simulink model "LateralController1"  (R2021a)
settings: Solver=VariableStepAuto  StartTime=0.0  StopTime=15  RelTol=1e-3
values from neighbouring files (symbols this model uses):
  CarWidth = 1.4    [controller_setup.m]
  Fyf = zeros(1,57)    [FyfLookup.m]
  ks = 0    [controller_setup.m]    (also in test.m)
  PredictionHorizon = 60    [controller_setup.m]
  SlipAngle = -SlipAngle    [FyfLookup.m]
  Ts = 0.05    [controller_setup.m]    (also in test.m = 0.1)
  Vx = 15    [controller_setup.m]    (also in test.m)
libraries: simulink_extras x4, mpclib x3, simulink x2, autolibshared x1
settings Model: Creator=dekunw  LastModifiedBy=chnwa
settings SolverCC: AlgebraicLoopSolver=TrustRegion
settings DebuggingCC: SFMachineParentedDataDiag=warning

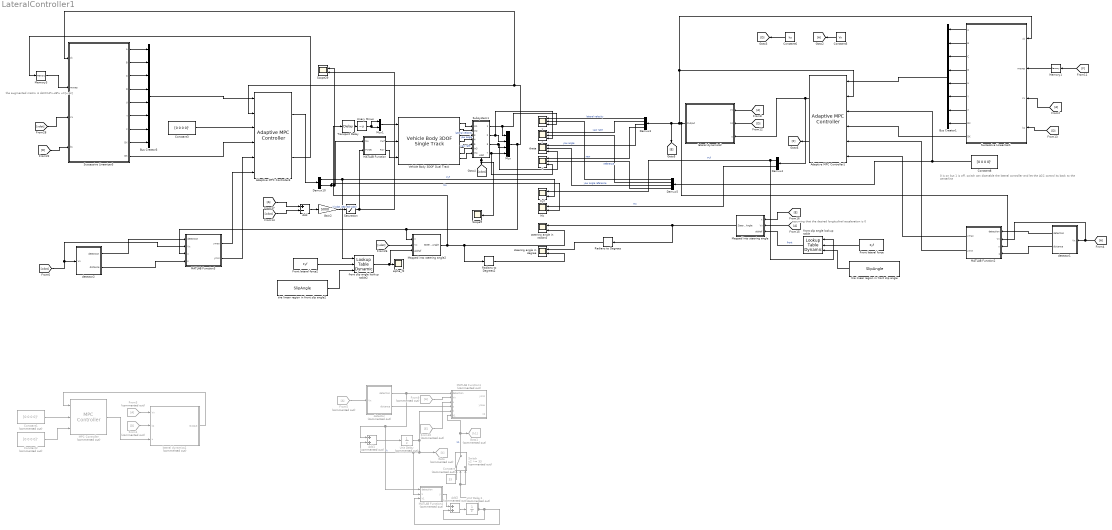
== system LateralController1 ==
  note: 0 is on but 1 is off. switch can disenable the lateral controller and let the ACC control its back to the centerline
  note: assuming that the desired longitudinal acceleration is 0
  note: the augmented matrix is dotX=A*x+B*u
      | u=[u;dc]
  Adaptive MPC Controller1 : mpclib/Adaptive MPC Controller  SCDEnableBlockLinearizationSpecification=on  mpcobj=mpc007  enable_value=0  updateMPCinCallerWorkspace=on  md_inport=on  mv_inport=off  uref_inport=off  return_cost=off  return_mvseq=on  return_qpstatus=off  return_xseq=off  return_state=off  return_ovseq=off  state_inport=off  isltv_plant=on  umin_inport=off  umax_inport=off  ymin_inport=on  ymax_inport=on  cc_inport=off  ywt_inport=off  uwt_inport=off  duwt_inport=off  rhoeps_inport=off  pm_inport=off  MaximumP=10  HorizonChoice=FixedHorizon  BlockDataType=double  SampleTimeInherited=off  switch_inport=off
  Adaptive MPC Controller3 : mpclib/Adaptive MPC Controller  SCDEnableBlockLinearizationSpecification=on  mpcobj=mpc007  enable_value=0  updateMPCinCallerWorkspace=on  md_inport=on  mv_inport=off  uref_inport=off  return_cost=off  return_mvseq=on  return_qpstatus=off  return_xseq=off  return_state=off  return_ovseq=off  state_inport=off  isltv_plant=on  umin_inport=off  umax_inport=off  ymin_inport=on  ymax_inport=on  cc_inport=off  ywt_inport=off  uwt_inport=off  duwt_inport=off  rhoeps_inport=off  pm_inport=off  MaximumP=10  HorizonChoice=FixedHorizon  BlockDataType=double  SampleTimeInherited=off  switch_inport=off
  Add : Sum  Inputs=+-
  Add1 : Sum  Commented=on
  Add2 : Sum  Commented=on
  Bus Creator1 : BusCreator  Inputs=8
  Bus Creator3 : BusCreator  Inputs=8
  Constant : Constant  Commented=on  Value=33
  Constant1 : Constant  Commented=on  Value=[0 0 0 0]'
  Constant2 : Constant  Commented=on  Value=[0 0 0 0]'
  Constant3 : Constant  Value=[0 0 0 0]'
  Constant5 : Constant  Value=Vx
  Constant6 : Constant  Value=ks
  Constant8 : Constant  Value=[0 0 0 0]'
  Demux10 : Demux  Outputs=2
  Demux3 : Demux
  Demux4 : Demux  Outputs=2
  Demux5 : Demux
  From1 : From  Commented=on  GotoTag=D
  From10 : From  Commented=on  GotoTag=E
  From3 : From  Commented=on
  From5 : From  Commented=on
  From9 : From  Commented=on
  Front lateral force : Constant  Value=Fyf
  Front lateral force2 : Constant  Value=Fyf
  Fyf : Scope  NumInputPorts=2
  Gain2 : Gain  Gain=5000
  Goto : Goto  Commented=on  GotoTag=k
  Goto1 : Goto  Commented=on  GotoTag=k1
  MATLAB Function : MATLAB Function  TreatAsAtomicUnit=on
  MATLAB Function1 : MATLAB Function  Commented=on  TreatAsAtomicUnit=on
  MATLAB Function2 : MATLAB Function  TreatAsAtomicUnit=on
  MATLAB Function3 : MATLAB Function  TreatAsAtomicUnit=on
  MATLAB Function4 : MATLAB Function  Commented=on  TreatAsAtomicUnit=on
  MPC Controller : mpclib/MPC Controller  Commented=on  SCDEnableBlockLinearizationSpecification=on  mpcobj=mpc007  is_multiple=0  enable_value=0  return_u0=off  updateMPCinCallerWorkspace=on  md_inport=on  mv_inport=off  uref_inport=off  return_cost=off  return_mvseq=off  return_qpstatus=off  return_xseq=off  return_state=off  return_ovseq=off  state_inport=off  umin_inport=off  umax_inport=off  ymin_inport=off  ymax_inport=off  cc_inport=off  ywt_inport=off  uwt_inport=off  duwt_inport=off  rhoeps_inport=off  pm_inport=off  MaximumP=10  HorizonChoice=FixedHorizon  n_ts=1  n_p=10  n_mv=1  n_md=1  n_ud=0  n_mo=1  n_uo=0  BlockDataType=double  SampleTimeInherited=off  switch_inport=off
  Mapped into steering angle : MATLAB Function  TreatAsAtomicUnit=on
  Mapped into steering angle2 : MATLAB Function  TreatAsAtomicUnit=on
  Memory1 : Memory
  Memory3 : Memory
  Mux : Mux
  Mux1 : Mux  Inputs=2
  Mx : Scope  NumInputPorts=2
  Radians to Degrees : simulink_extras/Transformations/Radians to Degrees
  Radians to Degrees2 : simulink_extras/Transformations/Radians to Degrees
  Saturation : Saturate  UpperLimit=1000  LowerLimit=-1000
  Scope29 : Scope  NumInputPorts=2
  Scope9 : Scope
  Subsystem1 : Subsystem
      settings: PortSchema="{\"entries\":[{\"content\":{\"sides\":[{\"content\":{\"connectorIds\":[\"In1\",\"In2\",\"In3\",\"In4\",\"In5\",\"In6\",\"In7\"]},\"type\":\"ConnectorPlacement.EquallySpacedRectSide\",\"uuid\":\"2d5dd366-cf22-44c4-87a2-f50a57f797af\"},{\"content\":{\"connectorIds\":[\"Out1\",\"Out2\",\"Out3\",\"Out4\"],\"side\":\"RIGHT\"},\"type\":\"ConnectorPlacement.EquallySpacedRectSide\",\"uuid\":\"241189f4-e75c-43e7-8a99-abbcb9c74d53\"},{\"content\":{\"connectorIds\":[],\"side\":\"TOP\"},\"type\":\"ConnectorPlacement.EquallySpacedRectSide\",\"uuid\":\"6b3eeef9-a362-4a78-9c5e-a6ce434eb6a9\"},{\"content\":{\"connectorIds\":[\"Out5\"],\"side\":\"BOTTOM\"},\"type\":\"ConnectorPlacement.EquallySpacedRectSide\",\"uuid\":\"31957e50-4414-4d01-b89b-c25b1ce64d81\"}]},\"type\":\"ConnectorPlacement.EquallySpacedConnector\",\"uuid\":\"717fdc80-cf7e-49a5-b82a-ccb520b44d0e\"}],\"packageUris\":[\"http://schema.mathworks.com/mf0/Connector/R2020b\"],\"version\":\"1.0\"}"
  Successive Linearizer1 : MATLAB Function  TreatAsAtomicUnit=on
  Successive Linearizer3 : MATLAB Function  TreatAsAtomicUnit=on
  Switch : Switch  Commented=on  Threshold=33
  Transport Delay : TransportDelay  DelayTime=Ts
  Unary Minus : UnaryMinus
  Unit Delay : UnitDelay  Commented=on  SampleTime=-1  HasFrameUpgradeWarning=on
  Unit Delay1 : UnitDelay  Commented=on  SampleTime=-1  HasFrameUpgradeWarning=on
  Vehicle Body 3DOF Dual Track : autolibshared/Vehicle Body 3DOF Single Track  trackMode=Dual  inputMode=External longitudinal forces  frontSteerMode=on  rearSteerMode=off  windMode=off  muMode=off  extFMode=off  extMMode=off  htchFMode=off  htchMMode=off  extXo=off  extpsio=off  extxdoto=off  extro=off  extYo=off  extTamb=off  extydoto=off  aMode=2  NF=2  NR=2  m=2272  a=1.11  b=1.67  h=0.35  dh=1  hh=0.2  X_o=0  xdot_o=Vx  CalphaMode=off  sigmaMode=on  d=0  hl=0  w=[CarWidth,CarWidth]  Cy_f=1.3e5  Cy_r=1.28e5  sigma_f=.1  sigma_r=.1  alpha_f_brk=[-.1 .1]  Cy_f_data=[-1.3e5 1.3e5]  alpha_r_brk=[-.1 .1]  Cy_r_data=[-1.3e5 1.3e5]  Y_o=0  ydot_o=0  Izz=4600  psi_o=0  r_o=0  Af=2  Cd=.3  Cl=.1  Cpm=.1  beta_w=[0:0.01:0.3]  Cs=[0:0.03:0.9]  Cym=[0:0.01:0.3]  Pabs=101325  Tair=273  g=9.81  mu=0.7  xdot_tol=.01  Fznom=5000  Fxtire_sat=7e4  Fytire_sat=7e4  longOff=0  latOff=0  vertOff=0  wrapAng=off
      settings: SourceProductBaseCode=PW,DR,MT,UV,VE
  Y : Scope  NumInputPorts=3
  alpha_f2 : Scope
  detector : Subsystem  Commented=on
  detector1 : Subsystem
  detector2 : Subsystem
  front slip angle lookup table : simulink/Lookup Tables/Lookup Table Dynamic  LookUpMeth=Interpolation-Use End Values  OutDataType=fixdt('double')  OutScaling=[]  OutputDataTypeScalingMode=Specify via dialog  OutDataTypeStr=double  DoSatur=off
  front slip angle lookup table2 : simulink/Lookup Tables/Lookup Table Dynamic  LookUpMeth=Interpolation-Use End Values  OutDataType=fixdt('double')  OutScaling=[]  OutputDataTypeScalingMode=Specify via dialog  OutDataTypeStr=double  DoSatur=off
  lateral dynamics1 : Subsystem  Commented=on
  lateral dynamics2 : Subsystem
  r : Scope  NumInputPorts=3
  steering angle in degree : Scope  NumInputPorts=2
  steering angle in radians : Scope  NumInputPorts=2
  theta : Scope  NumInputPorts=3
  tire linear region in front slip angle : Constant  Value=SlipAngle
  tire linear region in front slip angle2 : Constant  Value=SlipAngle
  v : Scope  NumInputPorts=3
  wires:
  Radians to Degrees/1 -> steering angle in degree/1
  Successive Linearizer3/4(D) -> Bus Creator3/4
  Mux/1 -> MATLAB Function3/3(x), Mapped into steering angle2/1(x), Successive Linearizer3/1(xk), Adaptive MPC Controller3/2
  Vehicle Body 3DOF Dual Track/3 -> Subsystem1/3(Input)  "lateral velocity"
  Successive Linearizer3/8(DX) -> Bus Creator3/8
  Vehicle Body 3DOF Dual Track/7 -> Subsystem1/7(In4)
  Vehicle Body 3DOF Dual Track/6 -> Subsystem1/6(In3)
  Adaptive MPC Controller3/2 -> Memory3/1
  Radians to Degrees2/1 -> steering angle in degree/2
  [xdot] -> Mapped into steering angle2/2(Vx)
  Successive Linearizer3/1(A) -> Bus Creator3/1
  Subsystem1/2(Output) -> r/3, Mux/2
  Successive Linearizer3/6(Y) -> Bus Creator3/6
  Gain2/1 -> Saturation/1  "k(xdot_desired-xdot)"
  Successive Linearizer1/8(DX) -> Bus Creator1/8
  Successive Linearizer3/7(X) -> Bus Creator3/7
  [A] -> Mapped into steering angle/2(Vx)
  Successive Linearizer3/2(B) -> Bus Creator3/2
  [D] -> Successive Linearizer3/4(ks)
  From9/1 -> MATLAB Function1/2(Vx)
  Add/1 -> Gain2/1
  tire linear region in front slip angle2/1 -> front slip angle lookup table2/3
  [A] -> Add/1
  Demux10/2 -> Scope29/1, MATLAB Function/1(Mx), Mx/2  "Mx"
  Subsystem1/5(xdot) -> Scope9/1, [xdot]
  [xdot] -> Successive Linearizer3/3(Vx)
  front slip angle lookup table/1 -> Mapped into steering angle/3(alphaf)  "front"
  [xdot] -> Add/2
  Transport Delay/1 -> Unary Minus/1
  Demux3/1 -> v/1  "lateral velocity"
  Constant3/1 -> Adaptive MPC Controller3/3
  Successive Linearizer1/9(DK) -> Adaptive MPC Controller1/4
  Subsystem1/3(Output1) -> theta/3, Mux/3
  Memory3/1 -> Successive Linearizer3/2(moves)
  Successive Linearizer1/7(X) -> Bus Creator1/7
  From10/1 -> MATLAB Function1/3(x)
  Vehicle Body 3DOF Dual Track/5 -> Subsystem1/5(Input2)  "yaw rate"
  Vehicle Body 3DOF Dual Track/2 -> Subsystem1/2(In2)
  Vehicle Body 3DOF Dual Track/1 -> Subsystem1/1(In1)
  Subsystem1/1(Output2) -> Mux/1, v/3
  Constant5/1 -> [A]
  Bus Creator3/1 -> Adaptive MPC Controller3/1
  Adaptive MPC Controller3/1 -> Demux10/1
  [D] -> Successive Linearizer1/4(ks)
  Front lateral force2/1 -> front slip angle lookup table2/2
  Constant6/1 -> [D]
  Demux5/3 -> theta/2  "yaw angle reference"
  Demux5/4 -> Y/2  "reference"
  Demux4/1 -> front slip angle lookup table/1, Fyf/1  "Fyf"
  Front lateral force/1 -> front slip angle lookup table/2
  Vehicle Body 3DOF Dual Track/4 -> Subsystem1/4(Input1)  "yaw angle"
  [E] -> Mapped into steering angle/1(x)
  Adaptive MPC Controller1/1 -> lateral dynamics2/3(u), Demux4/1
  tire linear region in front slip angle/1 -> front slip angle lookup table/3
  Successive Linearizer3/9(DK) -> Adaptive MPC Controller3/4
  Mapped into steering angle/1(SteeringAngle) -> steering angle in radians/1, Radians to Degrees/1
  Adaptive MPC Controller1/2 -> [F]
  Successive Linearizer1/6(Y) -> Bus Creator1/6
  Demux3/2 -> r/1  "yaw rate"
  Mapped into steering angle2/1(SteeringAngle) -> Radians to Degrees2/1, steering angle in radians/2, Transport Delay/1
  [D] -> lateral dynamics2/2(ks)
  Successive Linearizer3/5(U) -> Bus Creator3/5
  Successive Linearizer1/1(A) -> Bus Creator1/1
  Constant8/1 -> Demux5/1, Adaptive MPC Controller1/3
  Successive Linearizer1/3(C) -> Bus Creator1/3
  Successive Linearizer3/3(C) -> Bus Creator3/3
  Bus Creator1/1 -> Adaptive MPC Controller1/1
  Demux3/4 -> Y/1  "new"
  Memory1/1 -> Successive Linearizer1/2(moves)
  [A] -> lateral dynamics2/1(Vx)
  Successive Linearizer1/5(U) -> Bus Creator1/5
  Successive Linearizer1/2(B) -> Bus Creator1/2
  Demux5/2 -> r/2
  lateral dynamics2/1(Output) -> Demux3/1, [E], Successive Linearizer1/1(xk), Adaptive MPC Controller1/2, MATLAB Function2/3(x)
  Successive Linearizer1/4(D) -> Bus Creator1/4
  [F] -> Memory1/1
  Demux5/1 -> v/2
  Demux4/2 -> Mx/1  "Mx"
  [A] -> Successive Linearizer1/3(Vx)
  Demux3/3 -> theta/1  "yaw angle"
  Demux10/1 -> front slip angle lookup table2/1, Fyf/2  "Fyf"
  front slip angle lookup table2/1 -> Mapped into steering angle2/3(alphaf), alpha_f2/1
  MPC Controller/1 -> lateral dynamics1/3(u)
  From1/1 -> lateral dynamics1/2(ks)
  From3/1 -> lateral dynamics1/1(Vx)
  lateral dynamics1/1(Output) -> MPC Controller/1
  Constant1/1 -> MPC Controller/2
  Constant2/1 -> MPC Controller/3
  detector/1(detection) -> MATLAB Function4/1(detection), Add1/1, MATLAB Function1/1(detection)
  detector/2(distance) -> MATLAB Function1/4(s)
  From5/1 -> detector/1(Vx)
  Add1/1 -> Unit Delay/1
  Unit Delay/1 -> MATLAB Function1/5(k), MATLAB Function4/2(k), Add1/2, Goto/1  "k"
  MATLAB Function4/1(y) -> Add2/1
  Add2/1 -> Unit Delay1/1
  Unit Delay1/1 -> Switch/3, Switch/2, MATLAB Function4/3(k1), Add2/2
  Switch/1 -> Goto1/1, MATLAB Function1/6(k1)  "k1"
  Constant/1 -> Switch/1
  [A] -> MATLAB Function2/2(Vx), detector1/1(Vx)
  detector2/2(distance) -> MATLAB Function3/4(s)
  detector2/1(detection) -> MATLAB Function3/1(detection)
  [xdot] -> MATLAB Function3/2(Vx), detector2/1(Vx)
  MATLAB Function3/2(ymin) -> Adaptive MPC Controller3/5
  MATLAB Function3/1(ymax) -> Adaptive MPC Controller3/6
  MATLAB Function2/1(ymax) -> Adaptive MPC Controller1/6
  MATLAB Function2/2(ymin) -> Adaptive MPC Controller1/5
  detector1/2(distance) -> MATLAB Function2/4(s)
  detector1/1(detection) -> MATLAB Function2/1(detection)
  MATLAB Function/1(Fwf) -> Vehicle Body 3DOF Dual Track/2
  MATLAB Function/2(Fwr) -> Vehicle Body 3DOF Dual Track/3
  Mux1/1 -> Vehicle Body 3DOF Dual Track/1
  Subsystem1/4(Y) -> Y/3, Mux/4
  Saturation/1 -> MATLAB Function/2(Fxnet), Scope29/2
  Unary Minus/1 -> Mux1/2, Mux1/1

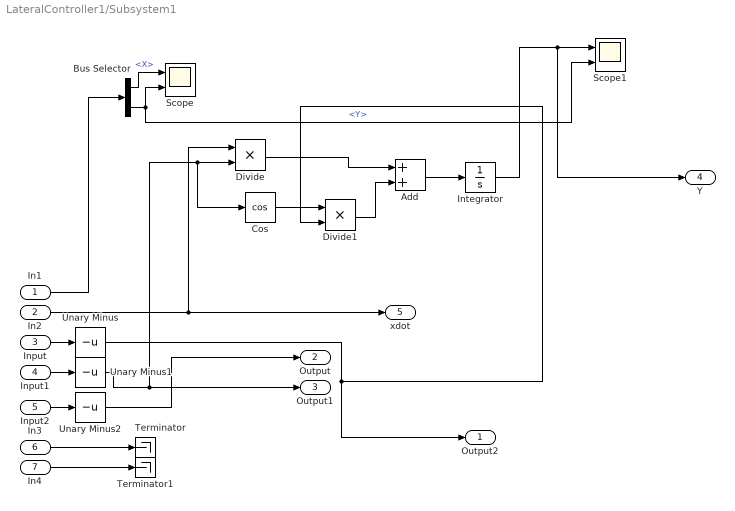
== system LateralController1/Subsystem1 ==
  In1 : Inport
  In2 : Inport  Port=2
  Input : Inport  Port=3
  Input1 : Inport  Port=4
  Input2 : Inport  Port=5
  In3 : Inport  Port=6
  In4 : Inport  Port=7
  Add : Sum
  Bus Selector : BusSelector  OutputSignals=InertFrm.Cg.Disp.X,InertFrm.Cg.Disp.Y
  Cos : Trigonometry  Operator=cos
  Divide : Product  Inputs=**
  Divide1 : Product  Inputs=**
  Integrator : Integrator
  Scope : Scope  NumInputPorts=2
  Scope1 : Scope  NumInputPorts=2
  Terminator : Terminator
  Terminator1 : Terminator
  Unary Minus : UnaryMinus
  Unary Minus1 : UnaryMinus
  Unary Minus2 : UnaryMinus
  Output2 : Outport
  Output : Outport  Port=2
  Output1 : Outport  Port=3
  Y : Outport  Port=4  SampleTime=Ts
  xdot : Outport  Port=5
  wires:
  In4/1 -> Terminator1/1
  In3/1 -> Terminator/1
  In2/1 -> xdot/1, Divide/1
  In1/1 -> Bus Selector/1
  Cos/1 -> Divide1/1
  Divide/1 -> Add/1
  Divide1/1 -> Add/2
  Add/1 -> Integrator/1
  Bus Selector/1 -> Scope/1  "<X>"
  Bus Selector/2 -> Scope/2, Scope1/2  "<Y>"
  Input2/1 -> Unary Minus2/1
  Integrator/1 -> Y/1, Scope1/1
  Input/1 -> Unary Minus/1
  Input1/1 -> Unary Minus1/1
  Unary Minus/1 -> Output2/1, Divide1/2
  Unary Minus1/1 -> Output1/1, Cos/1, Divide/2
  Unary Minus2/1 -> Output/1

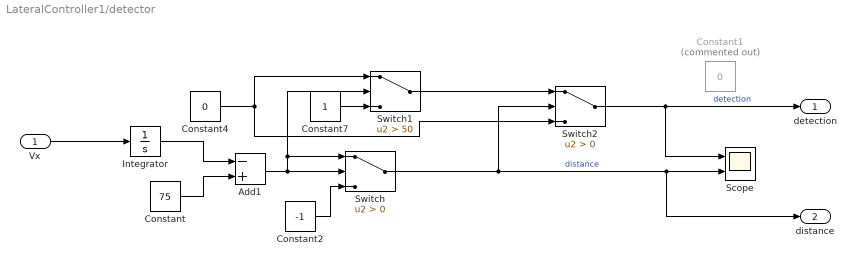
== system LateralController1/detector ==
  Vx : Inport
  Add1 : Sum  Inputs=-+
  Constant : Constant  Value=75
  Constant1 : Constant  Commented=on  Value=0
  Constant2 : Constant  Value=-1
  Constant4 : Constant  Value=0
  Constant7 : Constant
  Integrator : Integrator
  Scope : Scope  NumInputPorts=2
  Switch : Switch  Criteria=u2 > Threshold
  Switch1 : Switch  Criteria=u2 > Threshold  Threshold=50
  Switch2 : Switch  Criteria=u2 > Threshold
  detection : Outport
  distance : Outport  Port=2
  wires:
  Constant2/1 -> Switch/3
  Constant4/1 -> Switch2/3, Switch1/1
  Vx/1 -> Integrator/1
  Integrator/1 -> Add1/1
  Switch/1 -> Switch2/2, distance/1, Scope/2  "distance"
  Constant7/1 -> Switch1/3
  Add1/1 -> Switch1/2, Switch/1, Switch/2
  Switch1/1 -> Switch2/1
  Constant/1 -> Add1/2
  Switch2/1 -> detection/1, Scope/1  "detection"

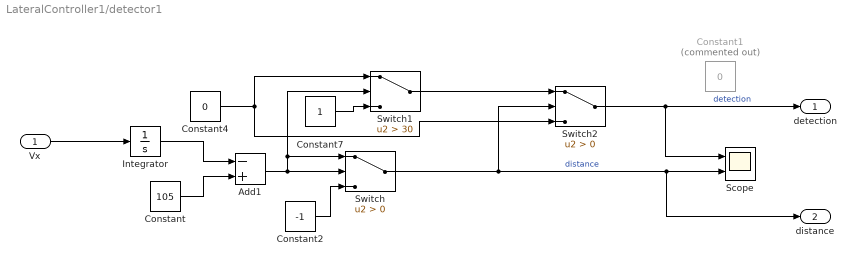
== system LateralController1/detector1 ==
  Vx : Inport
  Add1 : Sum  Inputs=-+
  Constant : Constant  Value=105
  Constant1 : Constant  Commented=on  Value=0
  Constant2 : Constant  Value=-1
  Constant4 : Constant  Value=0
  Constant7 : Constant
  Integrator : Integrator
  Scope : Scope  NumInputPorts=2
  Switch : Switch  Criteria=u2 > Threshold
  Switch1 : Switch  Criteria=u2 > Threshold  Threshold=30
  Switch2 : Switch  Criteria=u2 > Threshold
  detection : Outport
  distance : Outport  Port=2
  wires:
  Constant2/1 -> Switch/3
  Constant4/1 -> Switch2/3, Switch1/1
  Vx/1 -> Integrator/1
  Integrator/1 -> Add1/1
  Switch/1 -> Switch2/2, distance/1, Scope/2  "distance"
  Constant7/1 -> Switch1/3
  Add1/1 -> Switch1/2, Switch/1, Switch/2
  Switch1/1 -> Switch2/1
  Constant/1 -> Add1/2
  Switch2/1 -> Scope/1, detection/1  "detection"

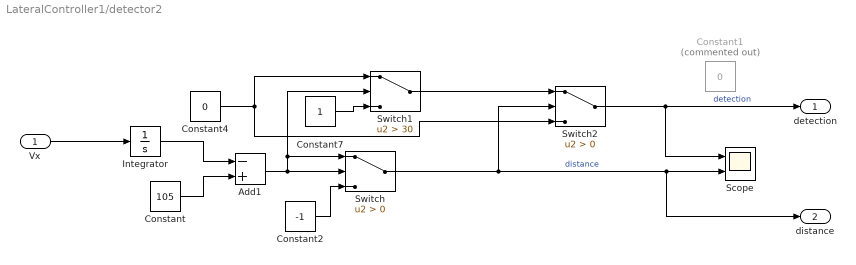
== system LateralController1/detector2 ==
  Vx : Inport
  Add1 : Sum  Inputs=-+
  Constant : Constant  Value=105
  Constant1 : Constant  Commented=on  Value=0
  Constant2 : Constant  Value=-1
  Constant4 : Constant  Value=0
  Constant7 : Constant
  Integrator : Integrator
  Scope : Scope  NumInputPorts=2
  Switch : Switch  Criteria=u2 > Threshold
  Switch1 : Switch  Criteria=u2 > Threshold  Threshold=30
  Switch2 : Switch  Criteria=u2 > Threshold
  detection : Outport
  distance : Outport  Port=2
  wires:
  Constant2/1 -> Switch/3
  Constant4/1 -> Switch2/3, Switch1/1
  Vx/1 -> Integrator/1
  Integrator/1 -> Add1/1
  Switch/1 -> Switch2/2, distance/1, Scope/2  "distance"
  Constant7/1 -> Switch1/3
  Add1/1 -> Switch1/2, Switch/1, Switch/2
  Switch1/1 -> Switch2/1
  Constant/1 -> Add1/2
  Switch2/1 -> Scope/1, detection/1  "detection"

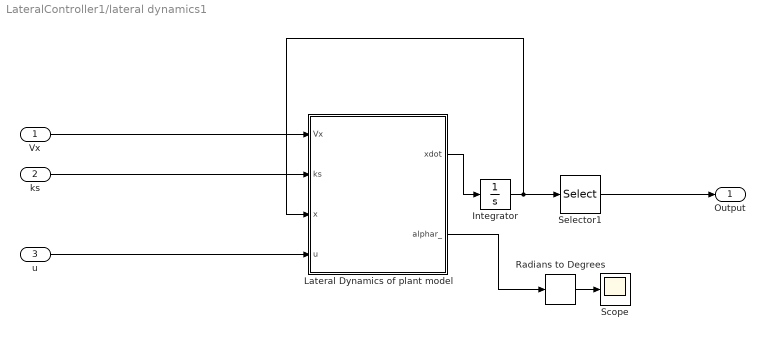
== system LateralController1/lateral dynamics1 ==
  Vx : Inport
  ks : Inport  Port=2
  u : Inport  Port=3
  Integrator : Integrator
  Lateral Dynamics of plant model : MATLAB Function  TreatAsAtomicUnit=on
  Radians to Degrees : simulink_extras/Transformations/Radians to Degrees
  Scope : Scope
  Selector1 : Selector  InputPortWidth=4  IndexOptions=Index vector (dialog)  Indices=[1 2 3 4]  OutputSizes=1
  Output : Outport
  wires:
  u/1 -> Lateral Dynamics of plant model/4(u)
  Lateral Dynamics of plant model/1(xdot) -> Integrator/1
  Integrator/1 -> Selector1/1, Lateral Dynamics of plant model/3(x)
  Selector1/1 -> Output/1
  ks/1 -> Lateral Dynamics of plant model/2(ks)
  Vx/1 -> Lateral Dynamics of plant model/1(Vx)
  Lateral Dynamics of plant model/2(alphar_) -> Radians to Degrees/1
  Radians to Degrees/1 -> Scope/1

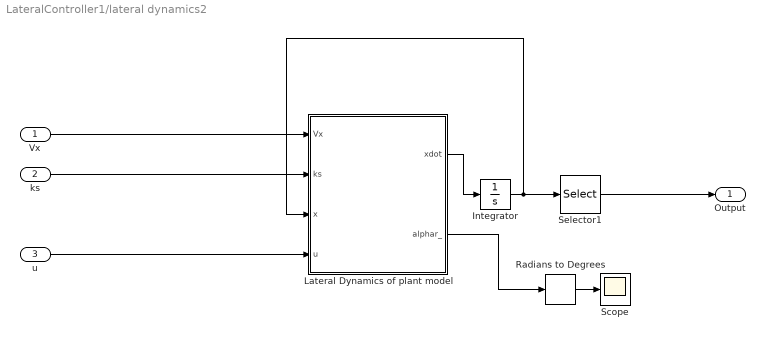
== system LateralController1/lateral dynamics2 ==
  Vx : Inport
  ks : Inport  Port=2
  u : Inport  Port=3
  Integrator : Integrator
  Lateral Dynamics of plant model : MATLAB Function  TreatAsAtomicUnit=on
  Radians to Degrees : simulink_extras/Transformations/Radians to Degrees
  Scope : Scope
  Selector1 : Selector  InputPortWidth=4  IndexOptions=Index vector (dialog)  Indices=[1 2 3 4]  OutputSizes=1
  Output : Outport
  wires:
  u/1 -> Lateral Dynamics of plant model/4(u)
  Lateral Dynamics of plant model/1(xdot) -> Integrator/1
  Integrator/1 -> Selector1/1, Lateral Dynamics of plant model/3(x)
  Selector1/1 -> Output/1
  ks/1 -> Lateral Dynamics of plant model/2(ks)
  Vx/1 -> Lateral Dynamics of plant model/1(Vx)
  Lateral Dynamics of plant model/2(alphar_) -> Radians to Degrees/1
  Radians to Degrees/1 -> Scope/1

== matlab function LateralController1/MATLAB Function4 ==
  data: detection input; y output; k input; k1 input
function y = fcn(detection,k, k1)

if (detection==0)&&(k==33)&&(k1<=33)
    y=1;
else
    y=0;
end

== matlab function LateralController1/Mapped into steering angle ==
  data: x input; Vx input; alphaf input; SteeringAngle output
function SteeringAngle = fcn(x,Vx, alphaf)

lf = 1.11;  % distance from front axle to the mass center

Vy = x(1); %lateral velocity
r = x(2);  %yaw rate
SteeringAngle = Vy/Vx+lf*r/Vx-alphaf;

== matlab function LateralController1/Mapped into steering angle2 ==
  data: x input; Vx input; alphaf input; SteeringAngle output
function SteeringAngle = fcn(x,Vx, alphaf)

lf = 1.11;  % distance from front axle to the mass center

Vy = x(1); %lateral velocity
r = x(2);  %yaw rate
SteeringAngle = Vy/Vx+lf*r/Vx-alphaf;

== matlab function LateralController1/Successive Linearizer3 ==
  data: A output size=[4,4,PredictionHorizon+1]; xk input size=[4,1]; moves input; B output size=[4,6,PredictionHorizon+1]; C output size=[4,4,PredictionHorizon+1]; D output size=[4,6,PredictionHorizon+1]; U output size=[6,1,PredictionHorizon+1]; Y output size=[4,1,PredictionHorizon+1]; X output size=[4,1,PredictionHorizon+1]; DX output size=[4,1,PredictionHorizon+1]; Vx input size=1; ks input; PredictionHorizon parameter size=1; DK output; Ts parameter size=1
function [A,B,C,D,U,Y,X,DX,DK] = fcn(xk,moves,Vx,ks, PredictionHorizon, Ts)
%sucessive updates the LTI plant model required by adaptive MPC controller

% LTV MPC requires p+1 linearizations from k to k+p
Steps = PredictionHorizon + 1; % having the number of Steps models
% Initialize outputs
A = zeros(4,4,Steps);
B = zeros(4,6,Steps);
C = zeros(4,4,Steps);
D = zeros(4,6,Steps);
U = zeros(6,1,Steps);
Y = zeros(4,1,Steps);
X = zeros(4,1,Steps);
DX = zeros(4,1,Steps);
DK = zeros(Steps,4); % the constant matrix in the model considered as measured disturbance

% Obtain time varying linear models via successive linearization
for ct = 1:Steps
    % since we don't have u(k) ... u(k+p) at the time of linearization,
    % previous optimal sequence u(k-1) ... u(k+p-1) is used instead.
    if ct>length(moves)
        uk = moves(Steps,:);
    else
        uk = moves(ct,:);
    end
    uk = uk';
    % analytical linearization (continuous time)
    [Ac, Bc, Cc, Dc, dc] = LateralDynamicsCT(Vx,ks,xk); % acquiring new characteristic matrix
    % convert A and B matrices from continuous time to discrete time
    % augmenting the model to be in the form of dotX=A*x+B*u while u=[u;dc]
    Aca = Ac;
    Bca = [Bc eye(4)];
    M = expm([[Aca Bca zeros(4,1)]*Ts;zeros(7,11)]);
    Ak = M(1:4,1:4);    %the discrete matrix A for augmented model
    Bk = M(1:4,5:10);   %the discrete matrix B for augmented model
    %store the state space matrix for ct time step
    A(:,:,ct) = Ak;
    B(:,:,ct) = Bk;
    C(:,:,ct) = Cc;
    D(:,:,ct) = [Dc,zeros(4,4)];  % always be zeros(4,6) in fact
    U(:,:,ct) = [uk;dc];          % measured disturbance dc is input as well
    Y(:,:,ct) = xk;               % output is all of the four states
    X(:,:,ct) = xk;               % four states
    DX(:,:,ct) = Ak*xk+Bk*[uk;dc]-xk;%the states increment
    DK(ct,:) = dc';               % disturbance in this step
    % next prediction step
    xk = DX(:,:,ct)+xk;           %update the states
end

%%%unrelated stuff
% ct= LTVu15_dist_Ts01.Model.Plant;
% dt = c2d(ct,Ts);
% LTVu15_dist_Ts01.Model.Plant = dt;

== matlab function LateralController1/MATLAB Function ==
  data: Fwf output size=[2,1]; Mx input; Fwr output size=[2,1]; Fxnet input
function [Fwf,Fwr] = fcn(Mx,Fxnet)

w = 1.4; % the width of the car

Fwf = zeros(2,1);
Fwr = zeros(2,1);

if Mx > 0
    Fwf(1) = Fxnet/2-Mx/w;
    Fwf(2) = Fxnet/2+0;
    Fwr(1) = -Mx/w;
    Fwr(2) = 0;
elseif Mx < 0
    Fwf(1) = Fxnet/2+0;
    Fwf(2) = Fxnet/2+Mx/w;
    Fwr(1) = 0;
    Fwr(2) = Mx/w;
else
    Fwf(1) = Fxnet/2+0;
    Fwf(2) = Fxnet/2+0;
    Fwr(1) = 0;
    Fwr(2) = 0;
end

== matlab function LateralController1/lateral dynamics1/Lateral Dynamics of plant model ==
  data: Vx input; ks input; x input; u input; xdot output; alphar_ output
function [xdot,alphar_] = fcn(Vx,ks, x, u)

%Plant Model parameters
m = 2272;   %mass
Iz = 4600;  %rotational inertia
lf = 1.11;  % distance from front axle to the mass center
lr = 1.67;  % distance from rear axle to the mass center
C_a = 1.3e5; % rear cornering stifness 

%Enviroment parameters
miu = 0.7; %frction cooeficient 0.7 for dry road and 0.4 for wet
g = 9.81; % gravity

Fz = m*g*lf/(lf+lr); % the load that beared by the rear tire

%calculate alpha
Vy = x(1); %lateral velocity
r = x(2);  %yaw rate
alphar_ = Vy/Vx-lr*r/Vx;   %calculate linearzing point

%tire model
threshold = atan(3*miu*Fz/C_a);
if abs(alphar_)<threshold
    Fyr_ = -C_a*tan(alphar_)+C_a^2/(3*miu*Fz)*abs(tan(alphar_))*tan(alphar_)-C_a^3/(27*miu^2*Fz^2)*tan(alphar_)^3;
    if alphar_>= 0
        Cr_ = -C_a*sec(alphar_)^2+C_a^2/(3*miu*Fz)*(2*sec(alphar_)^2*tan(alphar_))-C_a^3/(27*miu^2*Fz^2)*(3*tan(alphar_)^2*sec(alphar_)^2);
    else
        Cr_ = -C_a*sec(alphar_)^2-C_a^2/(3*miu*Fz)*(2*sec(alphar_)^2*tan(alphar_))-C_a^3/(27*miu^2*Fz^2)*(3*tan(alphar_)^2*sec(alphar_)^2);
    end
else
    Fyr_ = -miu*Fz*sign(alphar_);
    Cr_ = 0;
end

%Continuous-time model
Ac = [Cr_/(m*Vx) -lr*Cr_/(m*Vx)-Vx 0 0;
    -lr*Cr_/(Iz*Vx) lr^2*Cr_/(Iz*Vx) 0 0;
    0 1 0 0;
    1 0 Vx 0];
Bc = [1/m 0;
    lf/Iz 1/Iz;
    0 0;
    0 0];
dcc = [(Fyr_-Cr_*alphar_)/m;
    -lr*(Fyr_-Cr_*alphar_)/Iz;
    -Vx*ks;
    0];

% Cc =eye(4);
% Dc =zeros(4,2);
xdot = Ac*x + Bc*u +dcc;
% y = C*x + D*u;

== matlab function LateralController1/MATLAB Function2 ==
  data: detection input; ymax output size=[PredictionHorizon,4]; Vx input size=1; x input size=[4,1]; s input; PredictionHorizon parameter; ymin output size=[PredictionHorizon,4]; Ts parameter
function [ymax, ymin] = fcn(detection,Vx,x,s, PredictionHorizon, Ts)

miu = 0.7; %frction cooeficient 0.7 for dry road and 0.4 for wet
g = 9.81; % gravity
m = 2272;   %mass
lf = 1.11;  % distance from front axle to the mass center
lr = 1.67;  % distance from rear axle to the mass center
C_a = 1.3e5; % rear cornering stifness

Fz = m*g*lf/(lf+lr); % the load that beared by the rear tire

rmax = g*miu/Vx; %max yaw rate
threshold = atan(3*miu*Fz/C_a);

r = x(2);
vmax = lr*r+Vx*threshold;   %max lateral velocity
vmin = lr*r-Vx*threshold;   %min lateral velocity
k = round(s/Vx/Ts);
if k>PredictionHorizon
    k =PredictionHorizon;
elseif k<20
    k=20;
end

if detection == 1
    ymin1 = [vmin -rmax -pi/2 -10];%50m is the distance from which obstacle is detected
    ymax1 = [vmax rmax pi/2 10];
    ymin = repmat(ymin1,PredictionHorizon,1);
    ymax = repmat(ymax1,PredictionHorizon,1);
    k1=k-round(3/Vx/Ts);
    k2=k+round(3/Vx/Ts);
    if k1<1
        k1=1;
    end
    if k2>PredictionHorizon
        k2=PredictionHorizon;
    end
    ymin(k1:k2,4)=4;
    ymax(k1:k2,4)=6;
else
    ymin1 = [vmin -rmax -pi/2 -10];
    ymax1 = [vmax rmax pi/2 10];
    ymin = repmat(ymin1,PredictionHorizon,1);
    ymax = repmat(ymax1,PredictionHorizon,1);
end

== matlab function LateralController1/MATLAB Function3 ==
  data: detection input; ymax output size=[PredictionHorizon,4]; Vx input size=1; x input size=[4,1]; s input; PredictionHorizon parameter; ymin output size=[PredictionHorizon,4]; Ts parameter
function [ymax, ymin] = fcn(detection,Vx,x,s, PredictionHorizon, Ts)

miu = 0.7; %frction cooeficient 0.7 for dry road and 0.4 for wet
g = 9.81; % gravity
m = 2272;   %mass
lf = 1.11;  % distance from front axle to the mass center
lr = 1.67;  % distance from rear axle to the mass center
C_a = 1.3e5; % rear cornering stifness

Fz = m*g*lf/(lf+lr); % the load that beared by the rear tire

rmax = g*miu/Vx; %max yaw rate
threshold = atan(3*miu*Fz/C_a);

r = x(2);
vmax = lr*r+Vx*threshold;   %max lateral velocity
vmin = lr*r-Vx*threshold;   %min lateral velocity
k = round(s/Vx/Ts);
if k>PredictionHorizon
    k =PredictionHorizon;
elseif k<20
    k=20;
end

if detection == 1
    ymin1 = [vmin -rmax -pi/2 -10];%50m is the distance from which obstacle is detected
    ymax1 = [vmax rmax pi/2 10];
    ymin = repmat(ymin1,PredictionHorizon,1);
    ymax = repmat(ymax1,PredictionHorizon,1);
    k1=k-round(3/Vx/Ts);
    k2=k+round(3/Vx/Ts);
    if k1<1
        k1=1;
    end
    if k2>PredictionHorizon
        k2=PredictionHorizon;
    end
    ymin(k1:k2,4)=4;
    ymax(k1:k2,4)=6;
else
    ymin1 = [vmin -rmax -pi/2 -10];
    ymax1 = [vmax rmax pi/2 10];
    ymin = repmat(ymin1,PredictionHorizon,1);
    ymax = repmat(ymax1,PredictionHorizon,1);
end

== matlab function LateralController1/MATLAB Function1 ==
  data: detection input; ymin output; ymax output; Vx input; x input; s input; x4 output; k input; k1 input
function [ymin,ymax,x4] = fcn(detection,Vx,x,s,k,k1)

miu = 0.7; %frction cooeficient 0.7 for dry road and 0.4 for wet
g = 9.81; % gravity
m = 2272;   %mass
lf = 1.11;  % distance from front axle to the mass center
lr = 1.67;  % distance from rear axle to the mass center
C_a = 1.3e5; % rear cornering stifness

Fz = m*g*lf/(lf+lr); % the load that beared by the rear tire

rmax = g*miu/Vx; %max yaw rate
threshold = atan(3*miu*Fz/C_a);

r = x(2);
vmax = lr*r+Vx*threshold;   %max lateral velocity
vmin = lr*r-Vx*threshold;   %min lateral velocity

if (detection == 1)&&(s>0.1)
    ymin = [vmin -rmax -inf 4*k/30]';%50m is the distance from which obstacle is detected
    ymax = [vmax rmax inf 10]';
    x4 = ymin(4);
elseif ((detection == 0)&&(k==33))||((detection == 1)&&(k==32))
    ymin = [vmin -rmax -inf 4*(k-k1)/30]';%50m is the distance from which obstacle is detected
    ymax = [vmax rmax inf 10]';
    x4 = ymin(4);
else
    ymin = [vmin -rmax -pi/2 -10]';
    ymax = [vmax rmax pi/2 10]';
    x4 = 0;
end

== matlab function LateralController1/Successive Linearizer1 ==
  data: A output size=[4,4,PredictionHorizon+1]; xk input size=[4,1]; moves input; B output size=[4,6,PredictionHorizon+1]; C output size=[4,4,PredictionHorizon+1]; D output size=[4,6,PredictionHorizon+1]; U output size=[6,1,PredictionHorizon+1]; Y output size=[4,1,PredictionHorizon+1]; X output size=[4,1,PredictionHorizon+1]; DX output size=[4,1,PredictionHorizon+1]; Vx input size=1; ks input; PredictionHorizon parameter size=1; DK output; Ts parameter size=1
function [A,B,C,D,U,Y,X,DX,DK] = fcn(xk,moves,Vx,ks, PredictionHorizon, Ts)
%sucessive updates the LTI plant model required by adaptive MPC controller
% LTV MPC requires p+1 linearizations from k to k+p
Steps = PredictionHorizon + 1; % having the number of Steps models
% Initialize outputs
A = zeros(4,4,Steps);
B = zeros(4,6,Steps);
C = zeros(4,4,Steps);
D = zeros(4,6,Steps);
U = zeros(6,1,Steps);
Y = zeros(4,1,Steps);
X = zeros(4,1,Steps);
DX = zeros(4,1,Steps);
DK = zeros(Steps,4); % the constant matrix in the model considered as measured disturbance

% Obtain time varying linear models via successive linearization
for ct = 1:Steps
    % since we don't have u(k) ... u(k+p) at the time of linearization,
    % previous optimal sequence u(k-1) ... u(k+p-1) is used instead.
    if ct>length(moves)
        uk = moves(Steps,:);
    else
        uk = moves(ct,:);
    end
    uk = uk';
    % analytical linearization (continuous time)
    [Ac, Bc, Cc, Dc, dc] = LateralDynamicsCT(Vx,ks,xk); % acquiring new characteristic matrix
    % convert A and B matrices from continuous time to discrete time
    % augmenting the model to be in the form of dotX=A*x+B*u while u=[u;dc]
    Aca = Ac;
    Bca = [Bc eye(4)];
    M = expm([[Aca Bca zeros(4,1)]*Ts;zeros(7,11)]);
    Ak = M(1:4,1:4);    %the discrete matrix A for augmented model
    Bk = M(1:4,5:10);   %the discrete matrix B for augmented model
    %store the state space matrix for ct time step
    A(:,:,ct) = Ak;
    B(:,:,ct) = Bk;
    C(:,:,ct) = Cc;
    D(:,:,ct) = [Dc,zeros(4,4)];  % always be zeros(4,6) in fact
    U(:,:,ct) = [uk;dc];          % measured disturbance dc is input as well
    Y(:,:,ct) = xk;               % output is all of the four states
    X(:,:,ct) = xk;               % four states
    DX(:,:,ct) = Ak*xk+Bk*[uk;dc]-xk;%the states increment
    DK(ct,:) = dc';               % disturbance in this step
    % next prediction step
    xk = DX(:,:,ct)+xk;           %update the states
end

%%%unrelated stuff
% ct= LTVu15_dist_Ts01.Model.Plant;
% dt = c2d(ct,Ts);
% LTVu15_dist_Ts01.Model.Plant = dt;

== matlab function LateralController1/lateral dynamics2/Lateral Dynamics of plant model ==
  data: Vx input; ks input; x input; u input; xdot output; alphar_ output
function [xdot,alphar_] = fcn(Vx,ks, x, u)

%Plant Model parameters
m = 2272;   %mass
Iz = 4600;  %rotational inertia
lf = 1.11;  % distance from front axle to the mass center
lr = 1.67;  % distance from rear axle to the mass center
C_a = 1.3e5; % rear cornering stifness 

%Enviroment parameters
miu = 0.7; %frction cooeficient 0.7 for dry road and 0.4 for wet
g = 9.81; % gravity

Fz = m*g*lf/(lf+lr); % the load that beared by the rear tire

%calculate alpha
Vy = x(1); %lateral velocity
r = x(2);  %yaw rate
alphar_ = Vy/Vx-lr*r/Vx;   %calculate linearzing point

%tire model
threshold = atan(3*miu*Fz/C_a);
if abs(alphar_)<threshold
    Fyr_ = -C_a*tan(alphar_)+C_a^2/(3*miu*Fz)*abs(tan(alphar_))*tan(alphar_)-C_a^3/(27*miu^2*Fz^2)*tan(alphar_)^3;
    if alphar_>= 0
        Cr_ = -C_a*sec(alphar_)^2+C_a^2/(3*miu*Fz)*(2*sec(alphar_)^2*tan(alphar_))-C_a^3/(27*miu^2*Fz^2)*(3*tan(alphar_)^2*sec(alphar_)^2);
    else
        Cr_ = -C_a*sec(alphar_)^2-C_a^2/(3*miu*Fz)*(2*sec(alphar_)^2*tan(alphar_))-C_a^3/(27*miu^2*Fz^2)*(3*tan(alphar_)^2*sec(alphar_)^2);
    end
else
    Fyr_ = -miu*Fz*sign(alphar_);
    Cr_ = 0;
end

%Continuous-time model
Ac = [Cr_/(m*Vx) -lr*Cr_/(m*Vx)-Vx 0 0;
    -lr*Cr_/(Iz*Vx) lr^2*Cr_/(Iz*Vx) 0 0;
    0 1 0 0;
    1 0 Vx 0];
Bc = [1/m 0;
    lf/Iz 1/Iz;
    0 0;
    0 0];
dcc = [(Fyr_-Cr_*alphar_)/m;
    -lr*(Fyr_-Cr_*alphar_)/Iz;
    -Vx*ks;
    0];

% Cc =eye(4);
% Dc =zeros(4,2);
xdot = Ac*x + Bc*u +dcc;
% y = C*x + D*u;
